simulink model "rigLoggerMultipacket"  (R2012b)
settings: Solver=FixedStepDiscrete  StartTime=0.0  StopTime=10.0  FixedStep=0.001  RelTol=1e-3
undefined symbols (not defined in the file): macaddr, modelConstants
libraries: simulink x42, xpcethernetlib x29, xpcnetworkbufferlib x15, xpcutilitieslib x14, dspswit3 x14, dspmtrx3 x14, Lib_FileLoggerMultipacket x1
(part 2 of 5)

== system rigLoggerMultipacket/Neural2 Data & Format1/File Logger Data/File Logger Multipacket ==
  Packet Type : Inport
  FileName : Inport  Port=2
  Data : Inport  Port=3
  DataLen : Inport  Port=4
  transmitID : Inport  Port=5
  Enable : Inport  Port=6
  File Logger Wrapper : Subsystem
  MATLAB Function1 : MATLAB Function  TreatAsAtomicUnit=on
  Send Multipacket UDP : Subsystem  mask(Send Multipacket UDP Block){destMac=macaddr('ff:ff:ff:ff:ff:ff'), ID=2, prependHeader=off}
      mask prompts: destMac "Destination MAC:"; ID "Ethernet Device ID:"; prependHeader "Prepend 4-byte Header (uint16 length, uint16 checksum)"
      mask help: Splits a UDP packet into multiple pieces to be reassembled at the receiver
      mask TypeOptions ID: Ethernet Tx /ID
      mask Display:
      | disp([ 'Ethernet Tx ' num2str(ID)]);
      | port_label('input', 1, 'sourceIp');
      | port_label('input', 2, 'destIp');
      | port_label('input', 3, 'sourcePort');
      | port_label('input', 4, 'destPort');
      | port_label('input', 5, 'data (uint8)');
      | port_label('input', 6, 'transmitId (uint8)');
      | port_label('Enable','Enable')
  dIP : Constant  Value=modelConstants.filelogging.ip  OutDataTypeStr=uint8
  dPort : Constant  Value=modelConstants.filelogging.RECV_PORT  OutDataTypeStr=uint16
  sIP : Constant  Value=modelConstants.filelogging.xPCip  OutDataTypeStr=uint8
  sPort : Constant  Value=modelConstants.filelogging.SRC_PORT  OutDataTypeStr=uint16
  wires:
  transmitID/1 -> Send Multipacket UDP/6(transmitId)
  File Logger Wrapper/1(UDP Data) -> Send Multipacket UDP/5(Data)
  sIP/1 -> Send Multipacket UDP/1(sourceIP)
  dIP/1 -> Send Multipacket UDP/2(destIP)
  sPort/1 -> Send Multipacket UDP/3(sourcePort)
  dPort/1 -> Send Multipacket UDP/4(destPort)
  Enable/1 -> Send Multipacket UDP/Enable
  Data/1 -> File Logger Wrapper/3(Frame)
  DataLen/1 -> File Logger Wrapper/4(FrameSize)
  File Logger Wrapper/2(UDP Size) -> ?
  MATLAB Function1/1(y) -> File Logger Wrapper/2(FileName)
  Packet Type/1 -> File Logger Wrapper/1(Packet Type)
  FileName/1 -> MATLAB Function1/1(u)

== system rigLoggerMultipacket/Neural2 Data & Format1/File Logger Format/File Logger Multipacket ==
  Packet Type : Inport
  FileName : Inport  Port=2
  Data : Inport  Port=3
  DataLen : Inport  Port=4
  transmitID : Inport  Port=5
  Enable : Inport  Port=6
  File Logger Wrapper : Subsystem
  MATLAB Function1 : MATLAB Function  TreatAsAtomicUnit=on
  Send Multipacket UDP : Subsystem  mask(Send Multipacket UDP Block){destMac=macaddr('ff:ff:ff:ff:ff:ff'), ID=2, prependHeader=off}
      mask prompts: destMac "Destination MAC:"; ID "Ethernet Device ID:"; prependHeader "Prepend 4-byte Header (uint16 length, uint16 checksum)"
      mask help: Splits a UDP packet into multiple pieces to be reassembled at the receiver
      mask TypeOptions ID: Ethernet Tx /ID
      mask Display:
      | disp([ 'Ethernet Tx ' num2str(ID)]);
      | port_label('input', 1, 'sourceIp');
      | port_label('input', 2, 'destIp');
      | port_label('input', 3, 'sourcePort');
      | port_label('input', 4, 'destPort');
      | port_label('input', 5, 'data (uint8)');
      | port_label('input', 6, 'transmitId (uint8)');
      | port_label('Enable','Enable')
  dIP : Constant  Value=modelConstants.filelogging.ip  OutDataTypeStr=uint8
  dPort : Constant  Value=modelConstants.filelogging.RECV_PORT  OutDataTypeStr=uint16
  sIP : Constant  Value=modelConstants.filelogging.xPCip  OutDataTypeStr=uint8
  sPort : Constant  Value=modelConstants.filelogging.SRC_PORT  OutDataTypeStr=uint16
  wires:
  transmitID/1 -> Send Multipacket UDP/6(transmitId)
  File Logger Wrapper/1(UDP Data) -> Send Multipacket UDP/5(Data)
  sIP/1 -> Send Multipacket UDP/1(sourceIP)
  dIP/1 -> Send Multipacket UDP/2(destIP)
  sPort/1 -> Send Multipacket UDP/3(sourcePort)
  dPort/1 -> Send Multipacket UDP/4(destPort)
  Enable/1 -> Send Multipacket UDP/Enable
  Data/1 -> File Logger Wrapper/3(Frame)
  DataLen/1 -> File Logger Wrapper/4(FrameSize)
  File Logger Wrapper/2(UDP Size) -> ?
  MATLAB Function1/1(y) -> File Logger Wrapper/2(FileName)
  Packet Type/1 -> File Logger Wrapper/1(Packet Type)
  FileName/1 -> MATLAB Function1/1(u)

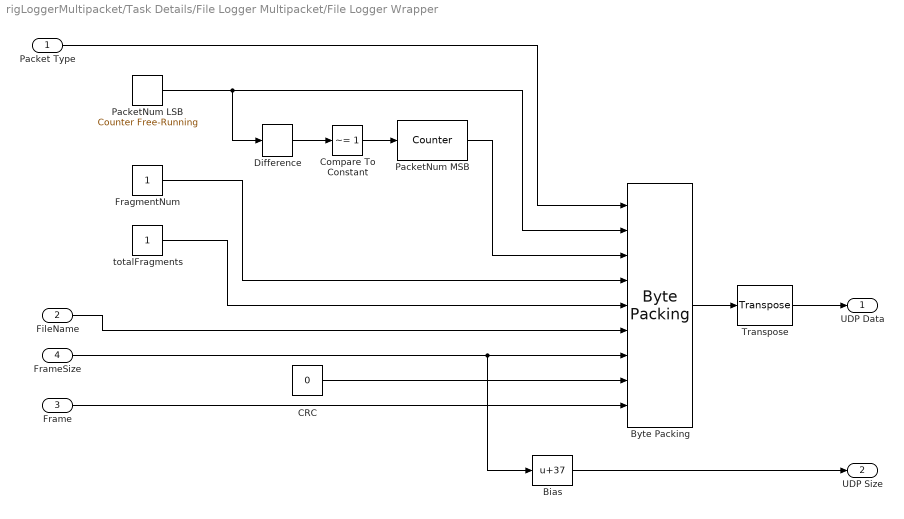
== system rigLoggerMultipacket/Task Details/File Logger Multipacket/File Logger Wrapper ==
  Packet Type : Inport
  FileName : Inport  Port=2
  Frame : Inport  Port=3
  FrameSize : Inport  Port=4
  Bias : Bias  Bias=37
  "Byte Packing " : xpcutilitieslib/Byte Packing   MaskPackedDataType=uint8  MaskUnpackedDataTypes={'boolean' 'uint32' 'uint32' 'uint8' 'uint8' 'uint8' 'uint16' 'uint32' 'uint8'}  MaskAlignment=1
  CRC : Constant  Value=0  OutDataTypeStr=uint32
  Compare To Constant : simulink/Logic and Bit Operations/Compare To Constant  relop=~=  const=1  OutDataTypeStr=uint8  ZeroCross=off
  Difference : simulink/Discrete/Difference  ICPrevInput=0  InputProcessing=Inherited  OutMin=[]  OutMax=[]  OutDataType=fixdt(1, 16)  OutScaling=2^-10  DoSatur=off
  FragmentNum : Constant  OutDataTypeStr=uint8
  PacketNum LSB : simulink/Sources/Counter Free-Running  NumBits=32  tsamp=-1
  PacketNum MSB : dspswit3/Counter  Direction=Up  CountEvent=Non-zero sample  CounterSize=32 bits  MaxCount=255  InitialCount=0  Output=Count  HitValue=32  ResetInput=off  SamplesPerFrame=1  Ts=1  CntDtype=uint32  HitDtype=Logical
  Transpose : dspmtrx3/Transpose  Hermitian=off  overflowFlag=off
  totalFragments : Constant  OutDataTypeStr=uint8
  UDP Data : Outport
  UDP Size : Outport  Port=2
  wires:
  Bias/1 -> UDP Size/1
  FileName/1 -> "Byte Packing "/6
  totalFragments/1 -> "Byte Packing "/5
  FragmentNum/1 -> "Byte Packing "/4
  PacketNum LSB/1 -> Difference/1, "Byte Packing "/2
  Packet Type/1 -> "Byte Packing "/1
  Difference/1 -> Compare To Constant/1
  Compare To Constant/1 -> PacketNum MSB/1
  PacketNum MSB/1 -> "Byte Packing "/3
  CRC/1 -> "Byte Packing "/8
  FrameSize/1 -> "Byte Packing "/7, Bias/1
  Frame/1 -> "Byte Packing "/9
  "Byte Packing "/1 -> Transpose/1
  Transpose/1 -> UDP Data/1

== system rigLoggerMultipacket/Task Details/File Logger Multipacket/Send Multipacket UDP ==
  sourceIP : Inport
  destIP : Inport  Port=2
  sourcePort : Inport  Port=3
  destPort : Inport  Port=4
  Data : Inport  Port=5  OutDataTypeStr=uint8
  transmitId : Inport  Port=6  OutDataTypeStr=uint8
  Enable : EnablePort
  "Ethernet Tx " : xpcethernetlib/Ethernet Tx   ID=2  SampleTime=-1
  For Iterator Subsystem : Subsystem  TreatAsAtomicUnit=on
  "Link " : xpcnetworkbufferlib/Link 
  MATLAB Function : MATLAB Function  TreatAsAtomicUnit=on
  MATLAB Function1 : MATLAB Function  TreatAsAtomicUnit=on
  TransmitBlockId1 : Constant  Value=uint8(prependHeader)  OutDataTypeStr=uint8
  wires:
  destPort/1 -> For Iterator Subsystem/7(destPort)
  sourcePort/1 -> For Iterator Subsystem/6(sourcePort)
  destIP/1 -> For Iterator Subsystem/5(destIP)
  sourceIP/1 -> For Iterator Subsystem/4(sourceIP)
  MATLAB Function/1(numPackets) -> For Iterator Subsystem/2(Num Packets)
  Data/1 -> MATLAB Function/1(in), For Iterator Subsystem/1(Data)
  transmitId/1 -> MATLAB Function1/1(transmitId)
  MATLAB Function1/1(datagramId) -> For Iterator Subsystem/3(Datagram Id)
  TransmitBlockId1/1 -> MATLAB Function/2(prependHeader)
  For Iterator Subsystem/1(NB Vector) -> "Link "/1
  "Link "/1 -> "Ethernet Tx "/1

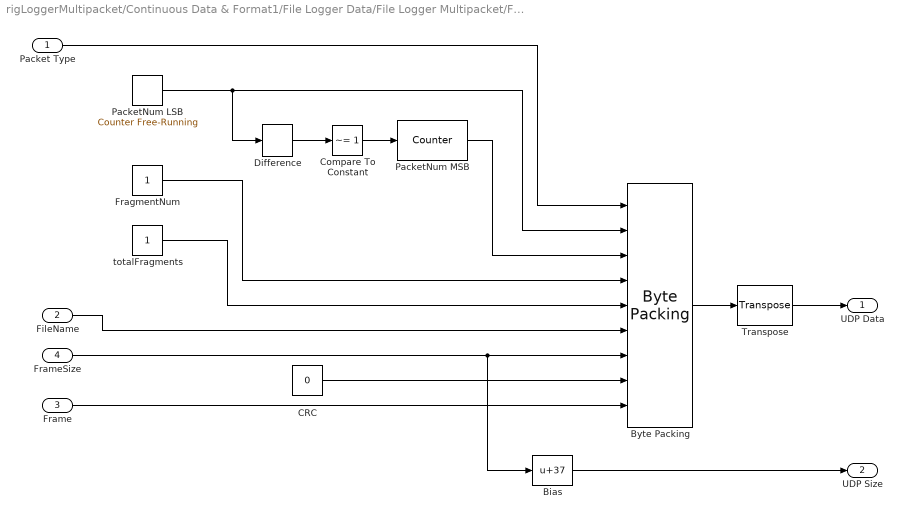
== system rigLoggerMultipacket/Continuous Data & Format1/File Logger Data/File Logger Multipacket/File Logger Wrapper ==
  Packet Type : Inport
  FileName : Inport  Port=2
  Frame : Inport  Port=3
  FrameSize : Inport  Port=4
  Bias : Bias  Bias=37
  "Byte Packing " : xpcutilitieslib/Byte Packing   MaskPackedDataType=uint8  MaskUnpackedDataTypes={'boolean' 'uint32' 'uint32' 'uint8' 'uint8' 'uint8' 'uint16' 'uint32' 'uint8'}  MaskAlignment=1
  CRC : Constant  Value=0  OutDataTypeStr=uint32
  Compare To Constant : simulink/Logic and Bit Operations/Compare To Constant  relop=~=  const=1  OutDataTypeStr=uint8  ZeroCross=off
  Difference : simulink/Discrete/Difference  ICPrevInput=0  InputProcessing=Inherited  OutMin=[]  OutMax=[]  OutDataType=fixdt(1, 16)  OutScaling=2^-10  DoSatur=off
  FragmentNum : Constant  OutDataTypeStr=uint8
  PacketNum LSB : simulink/Sources/Counter Free-Running  NumBits=32  tsamp=-1
  PacketNum MSB : dspswit3/Counter  Direction=Up  CountEvent=Non-zero sample  CounterSize=32 bits  MaxCount=255  InitialCount=0  Output=Count  HitValue=32  ResetInput=off  SamplesPerFrame=1  Ts=1  CntDtype=uint32  HitDtype=Logical
  Transpose : dspmtrx3/Transpose  Hermitian=off  overflowFlag=off
  totalFragments : Constant  OutDataTypeStr=uint8
  UDP Data : Outport
  UDP Size : Outport  Port=2
  wires:
  Bias/1 -> UDP Size/1
  FileName/1 -> "Byte Packing "/6
  totalFragments/1 -> "Byte Packing "/5
  FragmentNum/1 -> "Byte Packing "/4
  PacketNum LSB/1 -> Difference/1, "Byte Packing "/2
  Packet Type/1 -> "Byte Packing "/1
  Difference/1 -> Compare To Constant/1
  Compare To Constant/1 -> PacketNum MSB/1
  PacketNum MSB/1 -> "Byte Packing "/3
  CRC/1 -> "Byte Packing "/8
  FrameSize/1 -> "Byte Packing "/7, Bias/1
  Frame/1 -> "Byte Packing "/9
  "Byte Packing "/1 -> Transpose/1
  Transpose/1 -> UDP Data/1

== system rigLoggerMultipacket/Continuous Data & Format1/File Logger Data/File Logger Multipacket/Send Multipacket UDP ==
  sourceIP : Inport
  destIP : Inport  Port=2
  sourcePort : Inport  Port=3
  destPort : Inport  Port=4
  Data : Inport  Port=5  OutDataTypeStr=uint8
  transmitId : Inport  Port=6  OutDataTypeStr=uint8
  Enable : EnablePort
  "Ethernet Tx " : xpcethernetlib/Ethernet Tx   ID=2  SampleTime=-1
  For Iterator Subsystem : Subsystem  TreatAsAtomicUnit=on
  "Link " : xpcnetworkbufferlib/Link 
  MATLAB Function : MATLAB Function  TreatAsAtomicUnit=on
  MATLAB Function1 : MATLAB Function  TreatAsAtomicUnit=on
  TransmitBlockId1 : Constant  Value=uint8(prependHeader)  OutDataTypeStr=uint8
  wires:
  "Link "/1 -> "Ethernet Tx "/1
  For Iterator Subsystem/1(NB Vector) -> "Link "/1
  TransmitBlockId1/1 -> MATLAB Function/2(prependHeader)
  MATLAB Function1/1(datagramId) -> For Iterator Subsystem/3(Datagram Id)
  transmitId/1 -> MATLAB Function1/1(transmitId)
  Data/1 -> For Iterator Subsystem/1(Data), MATLAB Function/1(in)
  MATLAB Function/1(numPackets) -> For Iterator Subsystem/2(Num Packets)
  sourceIP/1 -> For Iterator Subsystem/4(sourceIP)
  destIP/1 -> For Iterator Subsystem/5(destIP)
  sourcePort/1 -> For Iterator Subsystem/6(sourcePort)
  destPort/1 -> For Iterator Subsystem/7(destPort)

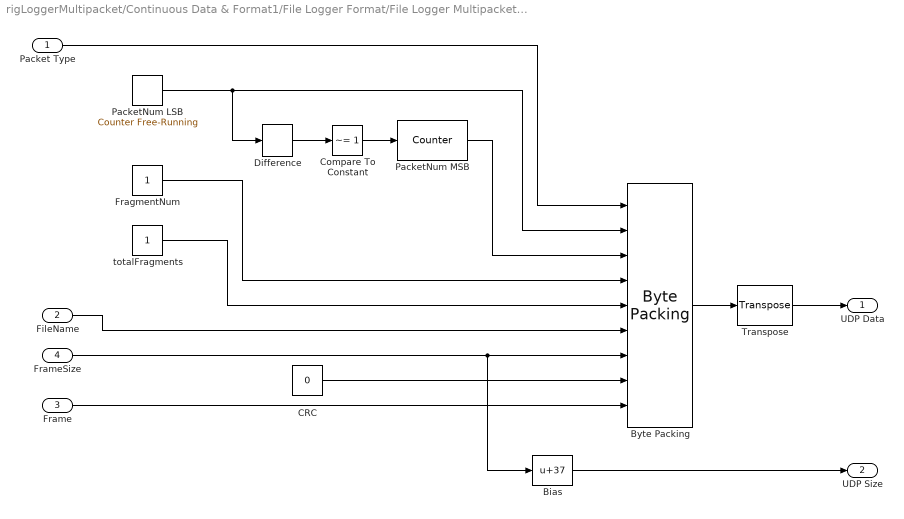
== system rigLoggerMultipacket/Continuous Data & Format1/File Logger Format/File Logger Multipacket/File Logger Wrapper ==
  Packet Type : Inport
  FileName : Inport  Port=2
  Frame : Inport  Port=3
  FrameSize : Inport  Port=4
  Bias : Bias  Bias=37
  "Byte Packing " : xpcutilitieslib/Byte Packing   MaskPackedDataType=uint8  MaskUnpackedDataTypes={'boolean' 'uint32' 'uint32' 'uint8' 'uint8' 'uint8' 'uint16' 'uint32' 'uint8'}  MaskAlignment=1
  CRC : Constant  Value=0  OutDataTypeStr=uint32
  Compare To Constant : simulink/Logic and Bit Operations/Compare To Constant  relop=~=  const=1  OutDataTypeStr=uint8  ZeroCross=off
  Difference : simulink/Discrete/Difference  ICPrevInput=0  InputProcessing=Inherited  OutMin=[]  OutMax=[]  OutDataType=fixdt(1, 16)  OutScaling=2^-10  DoSatur=off
  FragmentNum : Constant  OutDataTypeStr=uint8
  PacketNum LSB : simulink/Sources/Counter Free-Running  NumBits=32  tsamp=-1
  PacketNum MSB : dspswit3/Counter  Direction=Up  CountEvent=Non-zero sample  CounterSize=32 bits  MaxCount=255  InitialCount=0  Output=Count  HitValue=32  ResetInput=off  SamplesPerFrame=1  Ts=1  CntDtype=uint32  HitDtype=Logical
  Transpose : dspmtrx3/Transpose  Hermitian=off  overflowFlag=off
  totalFragments : Constant  OutDataTypeStr=uint8
  UDP Data : Outport
  UDP Size : Outport  Port=2
  wires:
  Bias/1 -> UDP Size/1
  FileName/1 -> "Byte Packing "/6
  totalFragments/1 -> "Byte Packing "/5
  FragmentNum/1 -> "Byte Packing "/4
  PacketNum LSB/1 -> Difference/1, "Byte Packing "/2
  Packet Type/1 -> "Byte Packing "/1
  Difference/1 -> Compare To Constant/1
  Compare To Constant/1 -> PacketNum MSB/1
  PacketNum MSB/1 -> "Byte Packing "/3
  CRC/1 -> "Byte Packing "/8
  FrameSize/1 -> "Byte Packing "/7, Bias/1
  Frame/1 -> "Byte Packing "/9
  "Byte Packing "/1 -> Transpose/1
  Transpose/1 -> UDP Data/1

== matlab function rigLoggerMultipacket/Neural Data & Format1/File Logger Data/File Logger Multipacket/Send Multipacket UDP/For Iterator
Subsystem/MATLAB Function1 ==
  data: idx input; vec output; in input
function vec = storeInVector(idx, in)
%#codegen

nPacketsMax = 15;

persistent pVec;
if isempty(pVec) || idx == 1
    pVec = repmat(in*0, nPacketsMax, 1);
end
if idx >= 1 && idx <= nPacketsMax
    pVec(idx) = in;
end

vec = pVec;

== matlab function rigLoggerMultipacket/Neural Data & Format1/File Logger Data/File Logger Multipacket/Send Multipacket UDP/MATLAB Function1 ==
  data: transmitId input uint8 size=1; datagramId output uint8 size=2
function datagramId = getDatagramId(transmitId)
%#codegen

% generates a unique id for this block, for this packet

persistent pId
if isempty(pId)
    pId = uint8(0);
else
    pId = pId + uint8(1);
end

datagramId = [transmitId; pId];

== matlab function rigLoggerMultipacket/Neural Data & Format1/File Logger Format/File Logger Multipacket/Send Multipacket UDP/For Iterator Subsystem/MATLAB Function ==
  data: data input uint8; numPackets input uint16 size=1; idxPacket input uint16 size=1; packetIP output uint8; lengthIP output uint16 size=1; sourceIP input uint8 size=4; sourcePort input uint16 size=1; destIP input uint8 size=4; destPort input uint16; datagramId input; prependHeader input
function [packetIP, lengthIP] = buildSubPacket(data, numPackets, idxPacket, sourceIP, sourcePort, destIP, destPort, datagramId, prependHeader)
%#codegen
% Creates a single UDP/IP packet that transmits one fragment of a possibly
% multi-fragment set of IP packets carrying the payload in data. idxPacket
% is the index of the fragment to send (1-indexed), out of num packets
% total fragments.
%
% Inputs:  
%   data : uint8 Nx1 or 1xN packet data vectors
%   numPackets, idxPacket : uint16 scalars
%   sourceIP, destIP : 1x4 uint8 of the IP (in address order)
%   sourcePort, destPort : uint16 port numbers
%   datagramId : uint16 scalar, unique id for this set of packets, for this timestep
%    that is used by the receiving IP stack to reassemble fragments
%   prependHeader : uint8 flag determining whether to prepend a 4 byte
%     header containing a 2 byte data length (excluding the header) and a 2
%     byte checksum (sum of bytes modulo 65536) of the data (excluding the 
%     header)
%
% Outputs:
%   packetIP : uint8 1500x1 IP packet to be passed into Create Ethernet
%     Packet block
%   lengthIP : uint16 scalar indicating the total length of packetIP
%     utilized, guaranteed to be even
% 
% Dan O'Shea, Paul Nuyujukian, Vikash Gilja
%

%% Initialize and return early if empty
packetIP = zeros(1500, 1, 'uint8');
lengthIP = uint16(0);

dataLength = numel(data);
if dataLength == 0
    return;
end

%% Build UDP subpacket

packetUDP = zeros(1480, 1, 'uint8');

% 1472 bytes per fragment
bytesPerFragment = uint16(1480);
headerUdpLength = uint16(8);
if prependHeader
    % 6 byte header on first packet containing '#u', 2 byte length, 2 byte checksum
    headerPreLength = uint16(4);
else
    headerPreLength = uint16(0);
end

headerLength = headerPreLength + headerUdpLength;

fragment = zeros(bytesPerFragment, 1, 'uint8');

% slice out the portion of data that goes in this packet
if idxPacket == 1
    byteStart = uint16(1);
    bytesThisFragment = bytesPerFragment - headerLength;
else
    % the first packet only graps 1480-8 bytes
    byteStart = uint16((idxPacket-uint16(1)) * bytesPerFragment - headerLength + uint16(1));
    bytesThisFragment = bytesPerFragment;
end

if byteStart > numel(data)
    % shouldn't happen, means idxPacket was too high for data
    return;
end
byteEnd = byteStart + bytesThisFragment - uint16(1);
% truncate fragment to data length
if byteEnd > numel(data)
    byteEnd = uint16(numel(data));
end
bytesThisFragment = byteEnd - byteStart + 1;

fragment(1:bytesThisFragment) = data(byteStart : byteEnd);

if idxPacket == 1
    if prependHeader
        headerPre = zeros(headerPreLength, 1, 'uint8');
        % 2 byte length
        headerPre(1:2) = typecast(uint16(numel(data)), 'uint8');
        % 2 byte modular checksum
        checksum = uint16(mod(sum(uint32(fragment)), uint32(65536)));
        headerPre(3:4) = typecast(checksum, 'uint8');
    else
        headerPre = [];
    end
        
    % include 8 byte udp header
    headerUdp = zeros(8, 1, 'uint8');
    FFFF = uint16(hex2dec('FFFF'));
    protocol = uint8(hex2dec('11'));
    length_BE = (typecast(uint16(numel(data)) + headerLength, 'uint8')); % flip to big endian
    length_BE = length_BE(end:-1:1);
    sourcePort_BE = (typecast(sourcePort, 'uint8'));
    sourcePort_BE = sourcePort_BE(end:-1:1);
    destPort_BE   = (typecast(destPort,   'uint8'));
    destPort_BE = destPort_BE(end:-1:1);
    headerUdp(1:8) = [sourcePort_BE destPort_BE length_BE uint8([0 0])];
    pseudoHeader = [sourceIP' destIP' uint8(0) protocol length_BE];
    
    if prependHeader
        % include 4 byte header in checksum
        if floor(double(numel(data)) / 2.0) ~= double(numel(data)) / 2.0
            % data is odd length, pad with zero byte
            checksumUdp = FFFF - uint16(mod( uint32(sum( typecast([pseudoHeader headerUdp' headerPre' data(:)' uint8(0)], 'uint16') )), uint32(FFFF) ));
        else
            checksumUdp = FFFF - uint16(mod( uint32(sum( typecast([pseudoHeader headerUdp' headerPre' data(:)'], 'uint16') )), uint32(FFFF) ));
        end
    else
        if floor(double(numel(data)) / 2.0) ~= double(numel(data)) / 2.0
            % data is odd length, pad with zero byte
            checksumUdp = FFFF - uint16(mod( uint32(sum( typecast([pseudoHeader headerUdp' data(:)' uint8(0)], 'uint16') )), uint32(FFFF) ));
        else
            checksumUdp = FFFF - uint16(mod( uint32(sum( typecast([pseudoHeader headerUdp' data(:)'], 'uint16') )), uint32(FFFF) ));
        end
    end
    headerUdp(7:8) = typecast(checksumUdp, 'uint8');

    % include custom 4 byte custom header with length and checksum
    if prependHeader
        lengthUDP = uint16(numel(headerUdp) + numel(headerPre) + bytesThisFragment);
        packetUDP(1:lengthUDP) = [headerUdp; headerPre; fragment(1:bytesThisFragment)];
    else
        % no header
        lengthUDP = uint16(numel(headerUdp) + bytesThisFragment);
        packetUDP(1:lengthUDP) = [headerUdp; fragment(1:bytesThisFragment)];
    end
else
    lengthUDP = uint16(bytesThisFragment);
    packetUDP(1:lengthUDP) = fragment(1:bytesThisFragment);
end

%% Build the fragment information that goes into IP header

% first 3 bits are 0, 1=DF, 2=More Fragments
% next 15 bits are length of fragment in bytes / 8
if idxPacket == 1
    fragmentWord = uint16(0);
else
    fragmentWord = (byteStart - uint16(1) + headerLength) / uint16(8);
end
if idxPacket < numPackets
    % set the more fragments bit
    fragmentWord = bitset(fragmentWord, 14);
end

% swap to big endian
fragmentBytes = typecast(fragmentWord, 'uint8')';
fragmentBytes = fragmentBytes([2;1]);

%% Build IP packet for this fragment

% make udp content length even
if floor(double(lengthUDP) / 2) ~= (double(lengthUDP) / 2)
    lengthUDP = lengthUDP + uint16(1);
end

% build IP header
lengthIP = lengthUDP + uint16(20);
version_IHL = uint8(69); % IPv4 and IP header length of 5
ToS = uint8(0); % no QOS on network

length_BE = (typecast(lengthIP, 'uint8')); % change to big endian
length_BE = length_BE(end:-1:1);

%ff = [ uint8(bin2dec('01000000')) 0 ]; % don't fragment packets
ff = fragmentBytes';
TTL = uint8(10); % ttl to 10 seconds/hops
protocol = uint8(hex2dec('11')); % UDP Protocol
headerIP = [ version_IHL ToS length_BE datagramId' ff TTL protocol 0 0 sourceIP' destIP'];

FFFF = uint16(hex2dec('FFFF'));
checksum = FFFF - uint16(mod( uint32(sum( typecast(headerIP, 'uint16') )), uint32(FFFF) ));
headerIP(11:12) = typecast(checksum, 'uint8');

% assemble the final packet
packetIP(1:lengthIP) = [ headerIP'; packetUDP(1:lengthUDP) ];

== matlab function rigLoggerMultipacket/Neural2 Data & Format1/File Logger Format/File Logger Multipacket/Send Multipacket UDP/For Iterator
Subsystem/MATLAB Function1 ==
  data: idx input; vec output; in input
function vec = storeInVector(idx, in)
%#codegen

nPacketsMax = 15;

persistent pVec;
if isempty(pVec) || idx == 1
    pVec = repmat(in*0, nPacketsMax, 1);
end
if idx >= 1 && idx <= nPacketsMax
    pVec(idx) = in;
end

vec = pVec;

== matlab function rigLoggerMultipacket/Neural2 Data & Format1/File Logger Format/File Logger Multipacket/Send Multipacket UDP/MATLAB Function ==
  data: in input; numPackets output uint16 size=1; prependHeader input
function numPackets = computeNumPackets(in, prependHeader)
%#codegen

% Assuming 1500 MTU, 1480 bytes per IP packet
% 8 bytes in udp header + 4 bytes in custom header if used, but only on the
% first fragment sent
if prependHeader
    headerLength = 8 + 6;
else
    headerLength = 8;
end
numPackets = uint16(ceil((double(numel(in))+headerLength) / 1480));

== matlab function rigLoggerMultipacket/Neural2 Data & Format1/File Logger Format/File Logger Multipacket/Send Multipacket UDP/MATLAB Function1 ==
  data: transmitId input uint8 size=1; datagramId output uint8 size=2
function datagramId = getDatagramId(transmitId)
%#codegen

% generates a unique id for this block, for this packet

persistent pId
if isempty(pId)
    pId = uint8(0);
else
    pId = pId + uint8(1);
end

datagramId = [transmitId; pId];

== matlab function rigLoggerMultipacket/DecoderC Data & Format1/File Logger Data/File Logger Multipacket/MATLAB Function1 ==
  data: u input; y output
function y = padFileName(u)

z = uint8(zeros(20, 1));

z(1:length(u)) = u;

y = z';

== matlab function rigLoggerMultipacket/DecoderC Data & Format1/File Logger Data/File Logger Multipacket/Send Multipacket UDP/For Iterator Subsystem/MATLAB Function ==
  data: data input uint8; numPackets input uint16 size=1; idxPacket input uint16 size=1; packetIP output uint8; lengthIP output uint16 size=1; sourceIP input uint8 size=4; sourcePort input uint16 size=1; destIP input uint8 size=4; destPort input uint16; datagramId input; prependHeader input
function [packetIP, lengthIP] = buildSubPacket(data, numPackets, idxPacket, sourceIP, sourcePort, destIP, destPort, datagramId, prependHeader)
%#codegen
% Creates a single UDP/IP packet that transmits one fragment of a possibly
% multi-fragment set of IP packets carrying the payload in data. idxPacket
% is the index of the fragment to send (1-indexed), out of num packets
% total fragments.
%
% Inputs:  
%   data : uint8 Nx1 or 1xN packet data vectors
%   numPackets, idxPacket : uint16 scalars
%   sourceIP, destIP : 1x4 uint8 of the IP (in address order)
%   sourcePort, destPort : uint16 port numbers
%   datagramId : uint16 scalar, unique id for this set of packets, for this timestep
%    that is used by the receiving IP stack to reassemble fragments
%   prependHeader : uint8 flag determining whether to prepend a 4 byte
%     header containing a 2 byte data length (excluding the header) and a 2
%     byte checksum (sum of bytes modulo 65536) of the data (excluding the 
%     header)
%
% Outputs:
%   packetIP : uint8 1500x1 IP packet to be passed into Create Ethernet
%     Packet block
%   lengthIP : uint16 scalar indicating the total length of packetIP
%     utilized, guaranteed to be even
% 
% Dan O'Shea, Paul Nuyujukian, Vikash Gilja
%

%% Initialize and return early if empty
packetIP = zeros(1500, 1, 'uint8');
lengthIP = uint16(0);

dataLength = numel(data);
if dataLength == 0
    return;
end

%% Build UDP subpacket

packetUDP = zeros(1480, 1, 'uint8');

% 1472 bytes per fragment
bytesPerFragment = uint16(1480);
headerUdpLength = uint16(8);
if prependHeader
    % 6 byte header on first packet containing '#u', 2 byte length, 2 byte checksum
    headerPreLength = uint16(4);
else
    headerPreLength = uint16(0);
end

headerLength = headerPreLength + headerUdpLength;

fragment = zeros(bytesPerFragment, 1, 'uint8');

% slice out the portion of data that goes in this packet
if idxPacket == 1
    byteStart = uint16(1);
    bytesThisFragment = bytesPerFragment - headerLength;
else
    % the first packet only graps 1480-8 bytes
    byteStart = uint16((idxPacket-uint16(1)) * bytesPerFragment - headerLength + uint16(1));
    bytesThisFragment = bytesPerFragment;
end

if byteStart > numel(data)
    % shouldn't happen, means idxPacket was too high for data
    return;
end
byteEnd = byteStart + bytesThisFragment - uint16(1);
% truncate fragment to data length
if byteEnd > numel(data)
    byteEnd = uint16(numel(data));
end
bytesThisFragment = byteEnd - byteStart + 1;

fragment(1:bytesThisFragment) = data(byteStart : byteEnd);

if idxPacket == 1
    if prependHeader
        headerPre = zeros(headerPreLength, 1, 'uint8');
        % 2 byte length
        headerPre(1:2) = typecast(uint16(numel(data)), 'uint8');
        % 2 byte modular checksum
        checksum = uint16(mod(sum(uint32(fragment)), uint32(65536)));
        headerPre(3:4) = typecast(checksum, 'uint8');
    else
        headerPre = [];
    end
        
    % include 8 byte udp header
    headerUdp = zeros(8, 1, 'uint8');
    FFFF = uint16(hex2dec('FFFF'));
    protocol = uint8(hex2dec('11'));
    length_BE = (typecast(uint16(numel(data)) + headerLength, 'uint8')); % flip to big endian
    length_BE = length_BE(end:-1:1);
    sourcePort_BE = (typecast(sourcePort, 'uint8'));
    sourcePort_BE = sourcePort_BE(end:-1:1);
    destPort_BE   = (typecast(destPort,   'uint8'));
    destPort_BE = destPort_BE(end:-1:1);
    headerUdp(1:8) = [sourcePort_BE destPort_BE length_BE uint8([0 0])];
    pseudoHeader = [sourceIP' destIP' uint8(0) protocol length_BE];
    
    if prependHeader
        % include 4 byte header in checksum
        if floor(double(numel(data)) / 2.0) ~= double(numel(data)) / 2.0
            % data is odd length, pad with zero byte
            checksumUdp = FFFF - uint16(mod( uint32(sum( typecast([pseudoHeader headerUdp' headerPre' data(:)' uint8(0)], 'uint16') )), uint32(FFFF) ));
        else
            checksumUdp = FFFF - uint16(mod( uint32(sum( typecast([pseudoHeader headerUdp' headerPre' data(:)'], 'uint16') )), uint32(FFFF) ));
        end
    else
        if floor(double(numel(data)) / 2.0) ~= double(numel(data)) / 2.0
            % data is odd length, pad with zero byte
            checksumUdp = FFFF - uint16(mod( uint32(sum( typecast([pseudoHeader headerUdp' data(:)' uint8(0)], 'uint16') )), uint32(FFFF) ));
        else
            checksumUdp = FFFF - uint16(mod( uint32(sum( typecast([pseudoHeader headerUdp' data(:)'], 'uint16') )), uint32(FFFF) ));
        end
    end
    headerUdp(7:8) = typecast(checksumUdp, 'uint8');

    % include custom 4 byte custom header with length and checksum
    if prependHeader
        lengthUDP = uint16(numel(headerUdp) + numel(headerPre) + bytesThisFragment);
        packetUDP(1:lengthUDP) = [headerUdp; headerPre; fragment(1:bytesThisFragment)];
    else
        % no header
        lengthUDP = uint16(numel(headerUdp) + bytesThisFragment);
        packetUDP(1:lengthUDP) = [headerUdp; fragment(1:bytesThisFragment)];
    end
else
    lengthUDP = uint16(bytesThisFragment);
    packetUDP(1:lengthUDP) = fragment(1:bytesThisFragment);
end

%% Build the fragment information that goes into IP header

% first 3 bits are 0, 1=DF, 2=More Fragments
% next 15 bits are length of fragment in bytes / 8
if idxPacket == 1
    fragmentWord = uint16(0);
else
    fragmentWord = (byteStart - uint16(1) + headerLength) / uint16(8);
end
if idxPacket < numPackets
    % set the more fragments bit
    fragmentWord = bitset(fragmentWord, 14);
end

% swap to big endian
fragmentBytes = typecast(fragmentWord, 'uint8')';
fragmentBytes = fragmentBytes([2;1]);

%% Build IP packet for this fragment

% make udp content length even
if floor(double(lengthUDP) / 2) ~= (double(lengthUDP) / 2)
    lengthUDP = lengthUDP + uint16(1);
end

% build IP header
lengthIP = lengthUDP + uint16(20);
version_IHL = uint8(69); % IPv4 and IP header length of 5
ToS = uint8(0); % no QOS on network

length_BE = (typecast(lengthIP, 'uint8')); % change to big endian
length_BE = length_BE(end:-1:1);

%ff = [ uint8(bin2dec('01000000')) 0 ]; % don't fragment packets
ff = fragmentBytes';
TTL = uint8(10); % ttl to 10 seconds/hops
protocol = uint8(hex2dec('11')); % UDP Protocol
headerIP = [ version_IHL ToS length_BE datagramId' ff TTL protocol 0 0 sourceIP' destIP'];

FFFF = uint16(hex2dec('FFFF'));
checksum = FFFF - uint16(mod( uint32(sum( typecast(headerIP, 'uint16') )), uint32(FFFF) ));
headerIP(11:12) = typecast(checksum, 'uint8');

% assemble the final packet
packetIP(1:lengthIP) = [ headerIP'; packetUDP(1:lengthUDP) ];

== matlab function rigLoggerMultipacket/DecoderD Data & Format1/File Logger Data/File Logger Multipacket/Send Multipacket UDP/For Iterator
Subsystem/MATLAB Function1 ==
  data: idx input; vec output; in input
function vec = storeInVector(idx, in)
%#codegen

nPacketsMax = 15;

persistent pVec;
if isempty(pVec) || idx == 1
    pVec = repmat(in*0, nPacketsMax, 1);
end
if idx >= 1 && idx <= nPacketsMax
    pVec(idx) = in;
end

vec = pVec;

== matlab function rigLoggerMultipacket/DecoderD Data & Format1/File Logger Data/File Logger Multipacket/Send Multipacket UDP/MATLAB Function ==
  data: in input; numPackets output uint16 size=1; prependHeader input
function numPackets = computeNumPackets(in, prependHeader)
%#codegen

% Assuming 1500 MTU, 1480 bytes per IP packet
% 8 bytes in udp header + 4 bytes in custom header if used, but only on the
% first fragment sent
if prependHeader
    headerLength = 8 + 6;
else
    headerLength = 8;
end
numPackets = uint16(ceil((double(numel(in))+headerLength) / 1480));

== matlab function rigLoggerMultipacket/DecoderD Data & Format1/File Logger Data/File Logger Multipacket/Send Multipacket UDP/MATLAB Function1 ==
  data: transmitId input uint8 size=1; datagramId output uint8 size=2
function datagramId = getDatagramId(transmitId)
%#codegen

% generates a unique id for this block, for this packet

persistent pId
if isempty(pId)
    pId = uint8(0);
else
    pId = pId + uint8(1);
end

datagramId = [transmitId; pId];

== matlab function rigLoggerMultipacket/DecoderD Data & Format1/File Logger Format/File Logger Multipacket/MATLAB Function1 ==
  data: u input; y output
function y = padFileName(u)

z = uint8(zeros(20, 1));

z(1:length(u)) = u;

y = z';

== matlab function rigLoggerMultipacket/DecoderD Data & Format1/File Logger Format/File Logger Multipacket/Send Multipacket UDP/For Iterator Subsystem/MATLAB Function ==
  data: data input uint8; numPackets input uint16 size=1; idxPacket input uint16 size=1; packetIP output uint8; lengthIP output uint16 size=1; sourceIP input uint8 size=4; sourcePort input uint16 size=1; destIP input uint8 size=4; destPort input uint16; datagramId input; prependHeader input
function [packetIP, lengthIP] = buildSubPacket(data, numPackets, idxPacket, sourceIP, sourcePort, destIP, destPort, datagramId, prependHeader)
%#codegen
% Creates a single UDP/IP packet that transmits one fragment of a possibly
% multi-fragment set of IP packets carrying the payload in data. idxPacket
% is the index of the fragment to send (1-indexed), out of num packets
% total fragments.
%
% Inputs:  
%   data : uint8 Nx1 or 1xN packet data vectors
%   numPackets, idxPacket : uint16 scalars
%   sourceIP, destIP : 1x4 uint8 of the IP (in address order)
%   sourcePort, destPort : uint16 port numbers
%   datagramId : uint16 scalar, unique id for this set of packets, for this timestep
%    that is used by the receiving IP stack to reassemble fragments
%   prependHeader : uint8 flag determining whether to prepend a 4 byte
%     header containing a 2 byte data length (excluding the header) and a 2
%     byte checksum (sum of bytes modulo 65536) of the data (excluding the 
%     header)
%
% Outputs:
%   packetIP : uint8 1500x1 IP packet to be passed into Create Ethernet
%     Packet block
%   lengthIP : uint16 scalar indicating the total length of packetIP
%     utilized, guaranteed to be even
% 
% Dan O'Shea, Paul Nuyujukian, Vikash Gilja
%

%% Initialize and return early if empty
packetIP = zeros(1500, 1, 'uint8');
lengthIP = uint16(0);

dataLength = numel(data);
if dataLength == 0
    return;
end

%% Build UDP subpacket

packetUDP = zeros(1480, 1, 'uint8');

% 1472 bytes per fragment
bytesPerFragment = uint16(1480);
headerUdpLength = uint16(8);
if prependHeader
    % 6 byte header on first packet containing '#u', 2 byte length, 2 byte checksum
    headerPreLength = uint16(4);
else
    headerPreLength = uint16(0);
end

headerLength = headerPreLength + headerUdpLength;

fragment = zeros(bytesPerFragment, 1, 'uint8');

% slice out the portion of data that goes in this packet
if idxPacket == 1
    byteStart = uint16(1);
    bytesThisFragment = bytesPerFragment - headerLength;
else
    % the first packet only graps 1480-8 bytes
    byteStart = uint16((idxPacket-uint16(1)) * bytesPerFragment - headerLength + uint16(1));
    bytesThisFragment = bytesPerFragment;
end

if byteStart > numel(data)
    % shouldn't happen, means idxPacket was too high for data
    return;
end
byteEnd = byteStart + bytesThisFragment - uint16(1);
% truncate fragment to data length
if byteEnd > numel(data)
    byteEnd = uint16(numel(data));
end
bytesThisFragment = byteEnd - byteStart + 1;

fragment(1:bytesThisFragment) = data(byteStart : byteEnd);

if idxPacket == 1
    if prependHeader
        headerPre = zeros(headerPreLength, 1, 'uint8');
        % 2 byte length
        headerPre(1:2) = typecast(uint16(numel(data)), 'uint8');
        % 2 byte modular checksum
        checksum = uint16(mod(sum(uint32(fragment)), uint32(65536)));
        headerPre(3:4) = typecast(checksum, 'uint8');
    else
        headerPre = [];
    end
        
    % include 8 byte udp header
    headerUdp = zeros(8, 1, 'uint8');
    FFFF = uint16(hex2dec('FFFF'));
    protocol = uint8(hex2dec('11'));
    length_BE = (typecast(uint16(numel(data)) + headerLength, 'uint8')); % flip to big endian
    length_BE = length_BE(end:-1:1);
    sourcePort_BE = (typecast(sourcePort, 'uint8'));
    sourcePort_BE = sourcePort_BE(end:-1:1);
    destPort_BE   = (typecast(destPort,   'uint8'));
    destPort_BE = destPort_BE(end:-1:1);
    headerUdp(1:8) = [sourcePort_BE destPort_BE length_BE uint8([0 0])];
    pseudoHeader = [sourceIP' destIP' uint8(0) protocol length_BE];
    
    if prependHeader
        % include 4 byte header in checksum
        if floor(double(numel(data)) / 2.0) ~= double(numel(data)) / 2.0
            % data is odd length, pad with zero byte
            checksumUdp = FFFF - uint16(mod( uint32(sum( typecast([pseudoHeader headerUdp' headerPre' data(:)' uint8(0)], 'uint16') )), uint32(FFFF) ));
        else
            checksumUdp = FFFF - uint16(mod( uint32(sum( typecast([pseudoHeader headerUdp' headerPre' data(:)'], 'uint16') )), uint32(FFFF) ));
        end
    else
        if floor(double(numel(data)) / 2.0) ~= double(numel(data)) / 2.0
            % data is odd length, pad with zero byte
            checksumUdp = FFFF - uint16(mod( uint32(sum( typecast([pseudoHeader headerUdp' data(:)' uint8(0)], 'uint16') )), uint32(FFFF) ));
        else
            checksumUdp = FFFF - uint16(mod( uint32(sum( typecast([pseudoHeader headerUdp' data(:)'], 'uint16') )), uint32(FFFF) ));
        end
    end
    headerUdp(7:8) = typecast(checksumUdp, 'uint8');

    % include custom 4 byte custom header with length and checksum
    if prependHeader
        lengthUDP = uint16(numel(headerUdp) + numel(headerPre) + bytesThisFragment);
        packetUDP(1:lengthUDP) = [headerUdp; headerPre; fragment(1:bytesThisFragment)];
    else
        % no header
        lengthUDP = uint16(numel(headerUdp) + bytesThisFragment);
        packetUDP(1:lengthUDP) = [headerUdp; fragment(1:bytesThisFragment)];
    end
else
    lengthUDP = uint16(bytesThisFragment);
    packetUDP(1:lengthUDP) = fragment(1:bytesThisFragment);
end

%% Build the fragment information that goes into IP header

% first 3 bits are 0, 1=DF, 2=More Fragments
% next 15 bits are length of fragment in bytes / 8
if idxPacket == 1
    fragmentWord = uint16(0);
else
    fragmentWord = (byteStart - uint16(1) + headerLength) / uint16(8);
end
if idxPacket < numPackets
    % set the more fragments bit
    fragmentWord = bitset(fragmentWord, 14);
end

% swap to big endian
fragmentBytes = typecast(fragmentWord, 'uint8')';
fragmentBytes = fragmentBytes([2;1]);

%% Build IP packet for this fragment

% make udp content length even
if floor(double(lengthUDP) / 2) ~= (double(lengthUDP) / 2)
    lengthUDP = lengthUDP + uint16(1);
end

% build IP header
lengthIP = lengthUDP + uint16(20);
version_IHL = uint8(69); % IPv4 and IP header length of 5
ToS = uint8(0); % no QOS on network

length_BE = (typecast(lengthIP, 'uint8')); % change to big endian
length_BE = length_BE(end:-1:1);

%ff = [ uint8(bin2dec('01000000')) 0 ]; % don't fragment packets
ff = fragmentBytes';
TTL = uint8(10); % ttl to 10 seconds/hops
protocol = uint8(hex2dec('11')); % UDP Protocol
headerIP = [ version_IHL ToS length_BE datagramId' ff TTL protocol 0 0 sourceIP' destIP'];

FFFF = uint16(hex2dec('FFFF'));
checksum = FFFF - uint16(mod( uint32(sum( typecast(headerIP, 'uint16') )), uint32(FFFF) ));
headerIP(11:12) = typecast(checksum, 'uint8');

% assemble the final packet
packetIP(1:lengthIP) = [ headerIP'; packetUDP(1:lengthUDP) ];

== system rigLoggerMultipacket/Continuous Data & Format1/File Logger Format/File Logger Multipacket/Send Multipacket UDP ==
  sourceIP : Inport
  destIP : Inport  Port=2
  sourcePort : Inport  Port=3
  destPort : Inport  Port=4
  Data : Inport  Port=5  OutDataTypeStr=uint8
  transmitId : Inport  Port=6  OutDataTypeStr=uint8
  Enable : EnablePort
  "Ethernet Tx " : xpcethernetlib/Ethernet Tx   ID=2  SampleTime=-1
  For Iterator Subsystem : Subsystem  TreatAsAtomicUnit=on
  "Link " : xpcnetworkbufferlib/Link 
  MATLAB Function : MATLAB Function  TreatAsAtomicUnit=on
  MATLAB Function1 : MATLAB Function  TreatAsAtomicUnit=on
  TransmitBlockId1 : Constant  Value=uint8(prependHeader)  OutDataTypeStr=uint8
  wires:
  "Link "/1 -> "Ethernet Tx "/1
  For Iterator Subsystem/1(NB Vector) -> "Link "/1
  TransmitBlockId1/1 -> MATLAB Function/2(prependHeader)
  MATLAB Function1/1(datagramId) -> For Iterator Subsystem/3(Datagram Id)
  transmitId/1 -> MATLAB Function1/1(transmitId)
  Data/1 -> For Iterator Subsystem/1(Data), MATLAB Function/1(in)
  MATLAB Function/1(numPackets) -> For Iterator Subsystem/2(Num Packets)
  sourceIP/1 -> For Iterator Subsystem/4(sourceIP)
  destIP/1 -> For Iterator Subsystem/5(destIP)
  sourcePort/1 -> For Iterator Subsystem/6(sourcePort)
  destPort/1 -> For Iterator Subsystem/7(destPort)

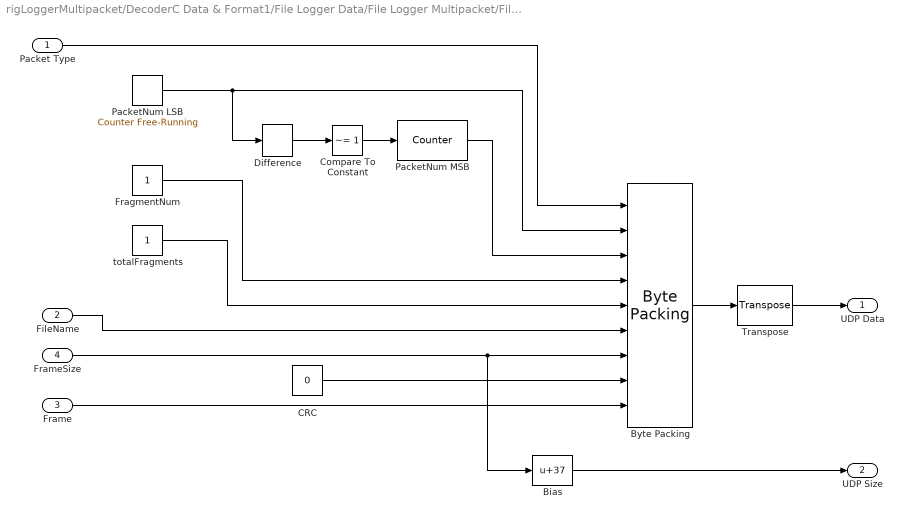
== system rigLoggerMultipacket/DecoderC Data & Format1/File Logger Data/File Logger Multipacket/File Logger Wrapper ==
  Packet Type : Inport
  FileName : Inport  Port=2
  Frame : Inport  Port=3
  FrameSize : Inport  Port=4
  Bias : Bias  Bias=37
  "Byte Packing " : xpcutilitieslib/Byte Packing   MaskPackedDataType=uint8  MaskUnpackedDataTypes={'boolean' 'uint32' 'uint32' 'uint8' 'uint8' 'uint8' 'uint16' 'uint32' 'uint8'}  MaskAlignment=1
  CRC : Constant  Value=0  OutDataTypeStr=uint32
  Compare To Constant : simulink/Logic and Bit Operations/Compare To Constant  relop=~=  const=1  OutDataTypeStr=uint8  ZeroCross=off
  Difference : simulink/Discrete/Difference  ICPrevInput=0  InputProcessing=Inherited  OutMin=[]  OutMax=[]  OutDataType=fixdt(1, 16)  OutScaling=2^-10  DoSatur=off
  FragmentNum : Constant  OutDataTypeStr=uint8
  PacketNum LSB : simulink/Sources/Counter Free-Running  NumBits=32  tsamp=-1
  PacketNum MSB : dspswit3/Counter  Direction=Up  CountEvent=Non-zero sample  CounterSize=32 bits  MaxCount=255  InitialCount=0  Output=Count  HitValue=32  ResetInput=off  SamplesPerFrame=1  Ts=1  CntDtype=uint32  HitDtype=Logical
  Transpose : dspmtrx3/Transpose  Hermitian=off  overflowFlag=off
  totalFragments : Constant  OutDataTypeStr=uint8
  UDP Data : Outport
  UDP Size : Outport  Port=2
  wires:
  Bias/1 -> UDP Size/1
  FileName/1 -> "Byte Packing "/6
  totalFragments/1 -> "Byte Packing "/5
  FragmentNum/1 -> "Byte Packing "/4
  PacketNum LSB/1 -> Difference/1, "Byte Packing "/2
  Packet Type/1 -> "Byte Packing "/1
  Difference/1 -> Compare To Constant/1
  Compare To Constant/1 -> PacketNum MSB/1
  PacketNum MSB/1 -> "Byte Packing "/3
  CRC/1 -> "Byte Packing "/8
  FrameSize/1 -> "Byte Packing "/7, Bias/1
  Frame/1 -> "Byte Packing "/9
  "Byte Packing "/1 -> Transpose/1
  Transpose/1 -> UDP Data/1

== system rigLoggerMultipacket/DecoderC Data & Format1/File Logger Data/File Logger Multipacket/Send Multipacket UDP ==
  sourceIP : Inport
  destIP : Inport  Port=2
  sourcePort : Inport  Port=3
  destPort : Inport  Port=4
  Data : Inport  Port=5  OutDataTypeStr=uint8
  transmitId : Inport  Port=6  OutDataTypeStr=uint8
  Enable : EnablePort
  "Ethernet Tx " : xpcethernetlib/Ethernet Tx   ID=2  SampleTime=-1
  For Iterator Subsystem : Subsystem  TreatAsAtomicUnit=on
  "Link " : xpcnetworkbufferlib/Link 
  MATLAB Function : MATLAB Function  TreatAsAtomicUnit=on
  MATLAB Function1 : MATLAB Function  TreatAsAtomicUnit=on
  TransmitBlockId1 : Constant  Value=uint8(prependHeader)  OutDataTypeStr=uint8
  wires:
  "Link "/1 -> "Ethernet Tx "/1
  For Iterator Subsystem/1(NB Vector) -> "Link "/1
  TransmitBlockId1/1 -> MATLAB Function/2(prependHeader)
  MATLAB Function1/1(datagramId) -> For Iterator Subsystem/3(Datagram Id)
  transmitId/1 -> MATLAB Function1/1(transmitId)
  Data/1 -> For Iterator Subsystem/1(Data), MATLAB Function/1(in)
  MATLAB Function/1(numPackets) -> For Iterator Subsystem/2(Num Packets)
  sourceIP/1 -> For Iterator Subsystem/4(sourceIP)
  destIP/1 -> For Iterator Subsystem/5(destIP)
  sourcePort/1 -> For Iterator Subsystem/6(sourcePort)
  destPort/1 -> For Iterator Subsystem/7(destPort)

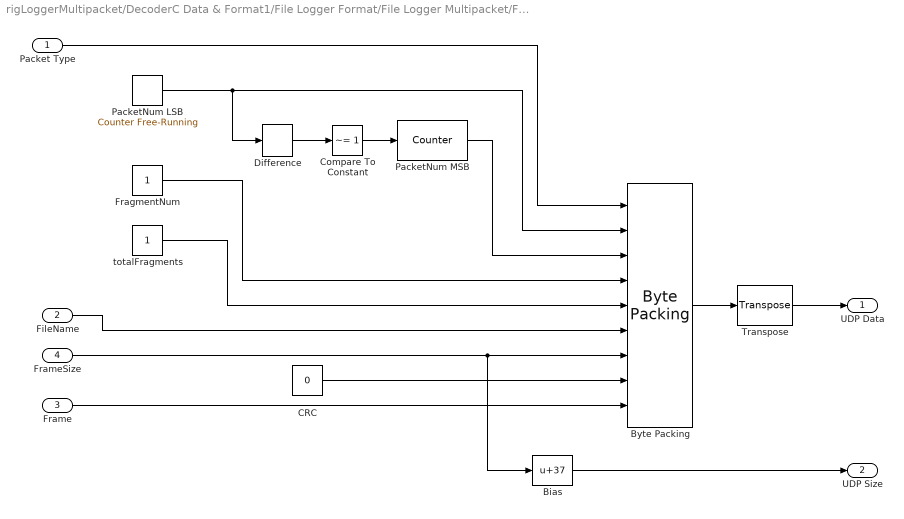
== system rigLoggerMultipacket/DecoderC Data & Format1/File Logger Format/File Logger Multipacket/File Logger Wrapper ==
  Packet Type : Inport
  FileName : Inport  Port=2
  Frame : Inport  Port=3
  FrameSize : Inport  Port=4
  Bias : Bias  Bias=37
  "Byte Packing " : xpcutilitieslib/Byte Packing   MaskPackedDataType=uint8  MaskUnpackedDataTypes={'boolean' 'uint32' 'uint32' 'uint8' 'uint8' 'uint8' 'uint16' 'uint32' 'uint8'}  MaskAlignment=1
  CRC : Constant  Value=0  OutDataTypeStr=uint32
  Compare To Constant : simulink/Logic and Bit Operations/Compare To Constant  relop=~=  const=1  OutDataTypeStr=uint8  ZeroCross=off
  Difference : simulink/Discrete/Difference  ICPrevInput=0  InputProcessing=Inherited  OutMin=[]  OutMax=[]  OutDataType=fixdt(1, 16)  OutScaling=2^-10  DoSatur=off
  FragmentNum : Constant  OutDataTypeStr=uint8
  PacketNum LSB : simulink/Sources/Counter Free-Running  NumBits=32  tsamp=-1
  PacketNum MSB : dspswit3/Counter  Direction=Up  CountEvent=Non-zero sample  CounterSize=32 bits  MaxCount=255  InitialCount=0  Output=Count  HitValue=32  ResetInput=off  SamplesPerFrame=1  Ts=1  CntDtype=uint32  HitDtype=Logical
  Transpose : dspmtrx3/Transpose  Hermitian=off  overflowFlag=off
  totalFragments : Constant  OutDataTypeStr=uint8
  UDP Data : Outport
  UDP Size : Outport  Port=2
  wires:
  Bias/1 -> UDP Size/1
  FileName/1 -> "Byte Packing "/6
  totalFragments/1 -> "Byte Packing "/5
  FragmentNum/1 -> "Byte Packing "/4
  PacketNum LSB/1 -> Difference/1, "Byte Packing "/2
  Packet Type/1 -> "Byte Packing "/1
  Difference/1 -> Compare To Constant/1
  Compare To Constant/1 -> PacketNum MSB/1
  PacketNum MSB/1 -> "Byte Packing "/3
  CRC/1 -> "Byte Packing "/8
  FrameSize/1 -> "Byte Packing "/7, Bias/1
  Frame/1 -> "Byte Packing "/9
  "Byte Packing "/1 -> Transpose/1
  Transpose/1 -> UDP Data/1

== system rigLoggerMultipacket/DecoderC Data & Format1/File Logger Format/File Logger Multipacket/Send Multipacket UDP ==
  sourceIP : Inport
  destIP : Inport  Port=2
  sourcePort : Inport  Port=3
  destPort : Inport  Port=4
  Data : Inport  Port=5  OutDataTypeStr=uint8
  transmitId : Inport  Port=6  OutDataTypeStr=uint8
  Enable : EnablePort
  "Ethernet Tx " : xpcethernetlib/Ethernet Tx   ID=2  SampleTime=-1
  For Iterator Subsystem : Subsystem  TreatAsAtomicUnit=on
  "Link " : xpcnetworkbufferlib/Link 
  MATLAB Function : MATLAB Function  TreatAsAtomicUnit=on
  MATLAB Function1 : MATLAB Function  TreatAsAtomicUnit=on
  TransmitBlockId1 : Constant  Value=uint8(prependHeader)  OutDataTypeStr=uint8
  wires:
  "Link "/1 -> "Ethernet Tx "/1
  For Iterator Subsystem/1(NB Vector) -> "Link "/1
  TransmitBlockId1/1 -> MATLAB Function/2(prependHeader)
  MATLAB Function1/1(datagramId) -> For Iterator Subsystem/3(Datagram Id)
  transmitId/1 -> MATLAB Function1/1(transmitId)
  Data/1 -> For Iterator Subsystem/1(Data), MATLAB Function/1(in)
  MATLAB Function/1(numPackets) -> For Iterator Subsystem/2(Num Packets)
  sourceIP/1 -> For Iterator Subsystem/4(sourceIP)
  destIP/1 -> For Iterator Subsystem/5(destIP)
  sourcePort/1 -> For Iterator Subsystem/6(sourcePort)
  destPort/1 -> For Iterator Subsystem/7(destPort)

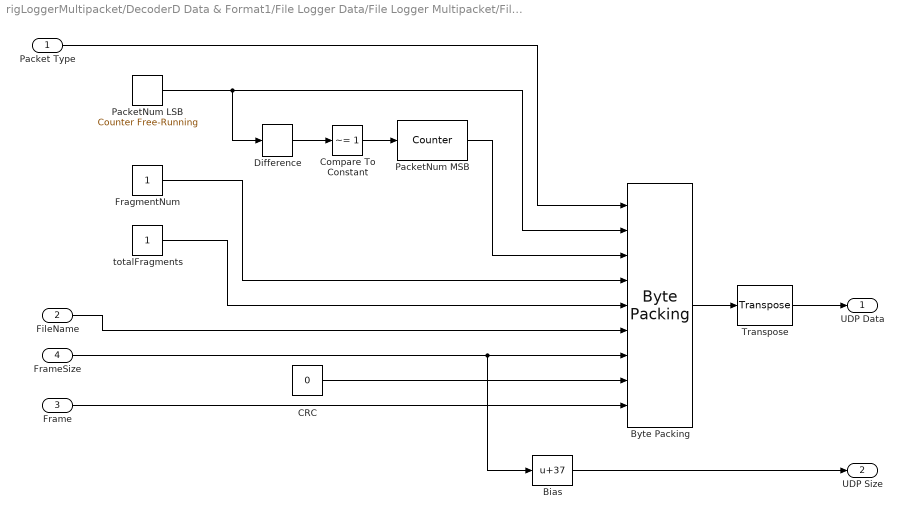
== system rigLoggerMultipacket/DecoderD Data & Format1/File Logger Data/File Logger Multipacket/File Logger Wrapper ==
  Packet Type : Inport
  FileName : Inport  Port=2
  Frame : Inport  Port=3
  FrameSize : Inport  Port=4
  Bias : Bias  Bias=37
  "Byte Packing " : xpcutilitieslib/Byte Packing   MaskPackedDataType=uint8  MaskUnpackedDataTypes={'boolean' 'uint32' 'uint32' 'uint8' 'uint8' 'uint8' 'uint16' 'uint32' 'uint8'}  MaskAlignment=1
  CRC : Constant  Value=0  OutDataTypeStr=uint32
  Compare To Constant : simulink/Logic and Bit Operations/Compare To Constant  relop=~=  const=1  OutDataTypeStr=uint8  ZeroCross=off
  Difference : simulink/Discrete/Difference  ICPrevInput=0  InputProcessing=Inherited  OutMin=[]  OutMax=[]  OutDataType=fixdt(1, 16)  OutScaling=2^-10  DoSatur=off
  FragmentNum : Constant  OutDataTypeStr=uint8
  PacketNum LSB : simulink/Sources/Counter Free-Running  NumBits=32  tsamp=-1
  PacketNum MSB : dspswit3/Counter  Direction=Up  CountEvent=Non-zero sample  CounterSize=32 bits  MaxCount=255  InitialCount=0  Output=Count  HitValue=32  ResetInput=off  SamplesPerFrame=1  Ts=1  CntDtype=uint32  HitDtype=Logical
  Transpose : dspmtrx3/Transpose  Hermitian=off  overflowFlag=off
  totalFragments : Constant  OutDataTypeStr=uint8
  UDP Data : Outport
  UDP Size : Outport  Port=2
  wires:
  Bias/1 -> UDP Size/1
  FileName/1 -> "Byte Packing "/6
  totalFragments/1 -> "Byte Packing "/5
  FragmentNum/1 -> "Byte Packing "/4
  PacketNum LSB/1 -> Difference/1, "Byte Packing "/2
  Packet Type/1 -> "Byte Packing "/1
  Difference/1 -> Compare To Constant/1
  Compare To Constant/1 -> PacketNum MSB/1
  PacketNum MSB/1 -> "Byte Packing "/3
  CRC/1 -> "Byte Packing "/8
  FrameSize/1 -> "Byte Packing "/7, Bias/1
  Frame/1 -> "Byte Packing "/9
  "Byte Packing "/1 -> Transpose/1
  Transpose/1 -> UDP Data/1

== system rigLoggerMultipacket/DecoderD Data & Format1/File Logger Data/File Logger Multipacket/Send Multipacket UDP ==
  sourceIP : Inport
  destIP : Inport  Port=2
  sourcePort : Inport  Port=3
  destPort : Inport  Port=4
  Data : Inport  Port=5  OutDataTypeStr=uint8
  transmitId : Inport  Port=6  OutDataTypeStr=uint8
  Enable : EnablePort
  "Ethernet Tx " : xpcethernetlib/Ethernet Tx   ID=2  SampleTime=-1
  For Iterator Subsystem : Subsystem  TreatAsAtomicUnit=on
  "Link " : xpcnetworkbufferlib/Link 
  MATLAB Function : MATLAB Function  TreatAsAtomicUnit=on
  MATLAB Function1 : MATLAB Function  TreatAsAtomicUnit=on
  TransmitBlockId1 : Constant  Value=uint8(prependHeader)  OutDataTypeStr=uint8
  wires:
  "Link "/1 -> "Ethernet Tx "/1
  For Iterator Subsystem/1(NB Vector) -> "Link "/1
  TransmitBlockId1/1 -> MATLAB Function/2(prependHeader)
  MATLAB Function1/1(datagramId) -> For Iterator Subsystem/3(Datagram Id)
  transmitId/1 -> MATLAB Function1/1(transmitId)
  Data/1 -> For Iterator Subsystem/1(Data), MATLAB Function/1(in)
  MATLAB Function/1(numPackets) -> For Iterator Subsystem/2(Num Packets)
  sourceIP/1 -> For Iterator Subsystem/4(sourceIP)
  destIP/1 -> For Iterator Subsystem/5(destIP)
  sourcePort/1 -> For Iterator Subsystem/6(sourcePort)
  destPort/1 -> For Iterator Subsystem/7(destPort)

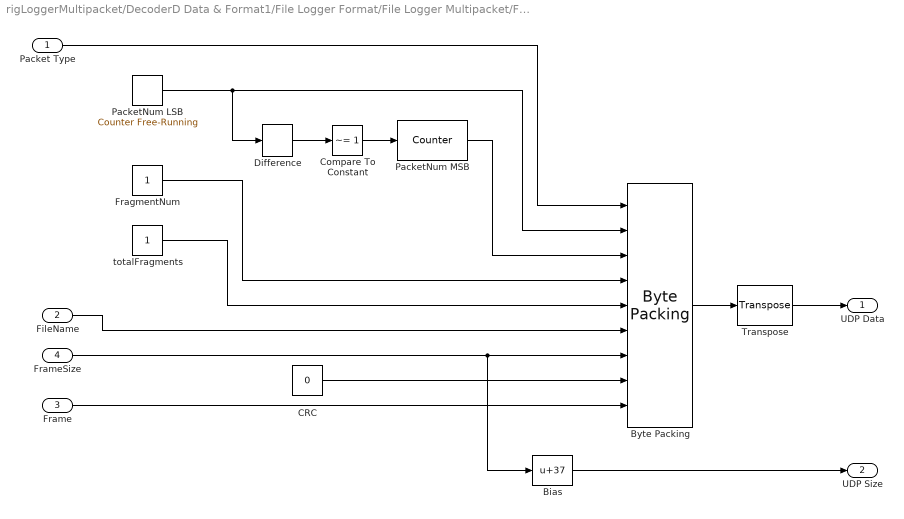
== system rigLoggerMultipacket/DecoderD Data & Format1/File Logger Format/File Logger Multipacket/File Logger Wrapper ==
  Packet Type : Inport
  FileName : Inport  Port=2
  Frame : Inport  Port=3
  FrameSize : Inport  Port=4
  Bias : Bias  Bias=37
  "Byte Packing " : xpcutilitieslib/Byte Packing   MaskPackedDataType=uint8  MaskUnpackedDataTypes={'boolean' 'uint32' 'uint32' 'uint8' 'uint8' 'uint8' 'uint16' 'uint32' 'uint8'}  MaskAlignment=1
  CRC : Constant  Value=0  OutDataTypeStr=uint32
  Compare To Constant : simulink/Logic and Bit Operations/Compare To Constant  relop=~=  const=1  OutDataTypeStr=uint8  ZeroCross=off
  Difference : simulink/Discrete/Difference  ICPrevInput=0  InputProcessing=Inherited  OutMin=[]  OutMax=[]  OutDataType=fixdt(1, 16)  OutScaling=2^-10  DoSatur=off
  FragmentNum : Constant  OutDataTypeStr=uint8
  PacketNum LSB : simulink/Sources/Counter Free-Running  NumBits=32  tsamp=-1
  PacketNum MSB : dspswit3/Counter  Direction=Up  CountEvent=Non-zero sample  CounterSize=32 bits  MaxCount=255  InitialCount=0  Output=Count  HitValue=32  ResetInput=off  SamplesPerFrame=1  Ts=1  CntDtype=uint32  HitDtype=Logical
  Transpose : dspmtrx3/Transpose  Hermitian=off  overflowFlag=off
  totalFragments : Constant  OutDataTypeStr=uint8
  UDP Data : Outport
  UDP Size : Outport  Port=2
  wires:
  Bias/1 -> UDP Size/1
  FileName/1 -> "Byte Packing "/6
  totalFragments/1 -> "Byte Packing "/5
  FragmentNum/1 -> "Byte Packing "/4
  PacketNum LSB/1 -> Difference/1, "Byte Packing "/2
  Packet Type/1 -> "Byte Packing "/1
  Difference/1 -> Compare To Constant/1
  Compare To Constant/1 -> PacketNum MSB/1
  PacketNum MSB/1 -> "Byte Packing "/3
  CRC/1 -> "Byte Packing "/8
  FrameSize/1 -> "Byte Packing "/7, Bias/1
  Frame/1 -> "Byte Packing "/9
  "Byte Packing "/1 -> Transpose/1
  Transpose/1 -> UDP Data/1
